simulink model "subsistema_mecanico"  (R2020a)
settings: Solver=VariableStepAuto  StartTime=0.0  StopTime=10.0  RelTol=1e-3
model workspace: external: MATLAB File D:\Ferran\Facultad\UNCuyo\Meca\Automática y Máquinas Eléctricas\Proyecto final\matlab2\parametros_y_especs\parametros_y_especif.m (data not in the file)
undefined symbols (not defined in the file): beq, Jeq, r
settings Model: Creator=Ferran  LastModifiedBy=Ferran

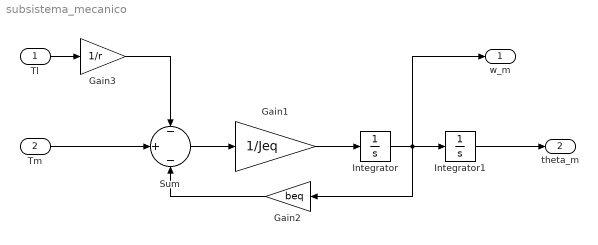
== system subsistema_mecanico ==
  Tl : Inport
  Tm : Inport  Port=2
  Gain1 : Gain  Gain=1/Jeq
  Gain2 : Gain  Gain=beq
  Gain3 : Gain  Gain=1/r
  Integrator : Integrator
  Integrator1 : Integrator
  Sum : Sum  Inputs=-|+|-
  w_m : Outport
  theta_m : Outport  Port=2
  wires:
  Tl/1 -> Gain3/1
  Tm/1 -> Sum/2
  Gain1/1 -> Integrator/1
  Sum/1 -> Gain1/1
  Gain2/1 -> Sum/3
  Integrator/1 -> w_m/1, Gain2/1, Integrator1/1
  Integrator1/1 -> theta_m/1
  Gain3/1 -> Sum/1
